simulink model "xeth"  (R2018a)
settings: Solver=VariableStepAuto  StartTime=0.0  StopTime=inf  RelTol=1e-3  EnableMultiTasking=on
undefined symbols (not defined in the file or in its folder): Part1, Part2, Part3, part4, RootGround, RootPart, taygap, xeth
libraries: mblibv1 x23, simulink x5
settings Model: Creator=phamn  LastModifiedBy=phamn
settings OptimizationCC: LifeSpan=inf
settings DebuggingCC: SFUnexpectedBacktrackingDiag=warning  SFNoUnconditionalDefaultTransitionDiag=warning  SFExecutionAtInitializationDiag=none
settings CodeAppCC: StateflowObjectComments=on
settings GRTTargetCC: TargetLangStandard=C89/C90 (ANSI)
settings ConfigComp: CovMetricSettings=dw  CovHtmlReporting=on  CovSaveCumulativeToWorkspaceVar=on  CovSaveSingleToWorkspaceVar=on  CovExternalEMLEnable=off
settings SimscapeCC: SimscapeNormalizeSystem=off
settings SimMechanicsCC: VisOnUpdateDiagram=on  VisDuringSimulation=on

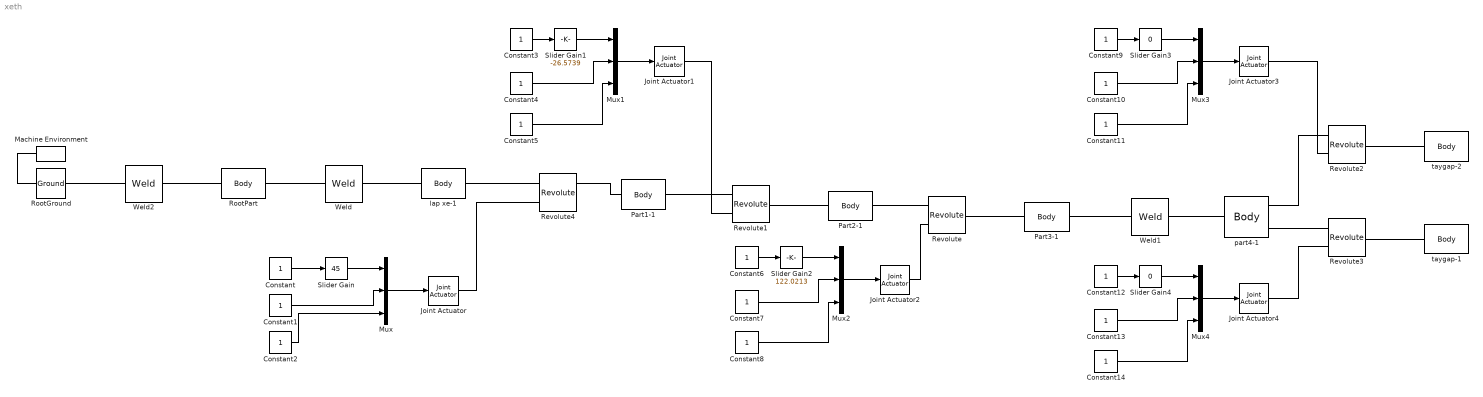
== system xeth ==
  Constant{,1..14} (15 alike) : Constant
  Joint Actuator{,1..4} (5 alike) : mblibv1/Sensors &  Actuators/Joint Actuator  UpdateFromCAD=off  PhysicalDomain=Mechanical  PortType=blob  ActuationStyle=Motion  AngleUnits=deg  ArcVelocityUnits=deg/s  ArcAccelerationUnits=deg/s^2  CoordPositionUnits=m  VelocityUnits=m/s  AccelerationUnits=m/s^2  ForceUnits=N  TorqueUnits=N*m  ActiveIO=on  Width=3  DialogClass=MechanicalActuatorBlock  Primitive=R1  ReferenceFrame=Absolute (World)
      settings: SourceProductName=Simscape  SourceProductBaseCode=SS
  Machine Environment : mblibv1/Bodies/Machine Environment  PortType=env  PhysicalDomain=Mechanical  DialogTemplateClass=MECH.MachineEnvironment  SyncWhenCopied=off  Gravity=[0 -9.81 0]  GravityUnits=m/s^2  GravityAsSignal=off  Dimensionality=Auto-detect  AnalysisType=Forward dynamics  LinearAssemblyTolerance=1e-3  LinearAssemblyToleranceUnits=m  AngularAssemblyTolerance=1e-3  AngularAssemblyToleranceUnits=rad  ConstraintSolverType=Stabilizing  ConstraintRelTolerance=1e-4  ConstraintAbsTolerance=1e-4  UseRobustSingularityHandling=off  RedundancyAnalysisToleranceType=Automatically select tolerance  RedundancyAnalysisTolerance=1e-14  StatePerturbationType=Fixed  PerturbationSize=1e-5  VisualizeMachine=on  BodyVisualizationType=Use model default body geometries  BodyColorSelMode=Use model default  DefaultBodyColor=[1 0 0]
      settings: SourceProductName=Simscape  SourceProductBaseCode=SS
  Mux{,1..4} (5 alike) : Mux  Inputs=3
  Part1-1 : mblibv1/Bodies/Body  LConnTagsString=CS3  RConnTagsString=CS2  UpdateFromCAD=on  PMImportedID=Part1-1  DialogClass=MechanicalBodyBlock  Mass=0.333703  MassUnits=kg  InertiaUnits=kg*m^2  Inertia=[0.00102628,0.000168229,6.01067e-10;0.000168229,0.000347488,-1.43807e-10;6.01067e-10,-1.43807e-10,0.000952025]  Shape=Cylinder  ShapeDims=[1 1]  ShapeUnits=m  ShapeUse=false  Density=1  DensityUnits=kg/m^3  DensityUse=false  GraphicsMode=GFXFILE  GraphicsFileName=xeth - Part1-1.STL  BodyColorSelMode=COLORPALETTE  BodyColor=[0.690196;0.658824;0.639216]  AttachedToCS=CS1  CG=Right$CG$[-0.0199579 0.0681608 0.0476382]$WORLD$WORLD$m$[-0.547791 0 0.836615;0 1 0;-0.836615 0 -0.547791]$3x3 Transform$rad$WORLD$false$Part1-1::CG(AUTOGEN)  WorkingFrames=Right$CS1$[-0.00787331 0.16628 0.0660944]$WORLD$WORLD$m$[-0.547791 0 0.836615;0 1 0;-0.836615 0 -0.547791]$3x3 Transform$rad$WORLD$false$Part1-1::CS1(AUTOGEN)#Right$CS2$[0.0109505 0.16628 0.0537691]$WORLD$WORLD$m$[1 0 0;0 1 0;0 0 1]$3x3 Transform$rad$WORLD$true$Part1-1:-:Part2-1::Part1-1(AUTOGEN)#Left$CS3$[-0.024307 0.02628 0.0409959]$WORLD$WORLD$m$[1 0 0;0 1 0;0 0 1]$3x3 Transform$rad$WORLD$true$Part1-1:-:lap xe-1::Part1-1(AUTOGEN)  CGPos=[-0.0199579 0.0681608 0.0476382]  CGRot=[-0.547791 0 0.836615;0 1 0;-0.836615 0 -0.547791]  CS0Pos=[]  CS0Rot=[]  CS1Pos=[-0.00787331 0.16628 0.0660944]  CS1Rot=[-0.547791 0 0.836615;0 1 0;-0.836615 0 -0.547791]  CS2Pos=[0.0109505 0.16628 0.0537691]  CS2Rot=[1 0 0;0 1 0;0 0 1]  CS3Pos=[-0.024307 0.02628 0.0409959]  CS3Rot=[1 0 0;0 1 0;0 0 1]  CS4Pos=[]  CS4Rot=[]  CS5Pos=[]  CS5Rot=[]  CS6Pos=[]  CS6Rot=[]  CS7Pos=[]  CS7Rot=[]  CS8Pos=[]  CS8Rot=[]  CS9Pos=[]  CS9Rot=[]  CS10Pos=[]  CS10Rot=[]  CS11Pos=[]  CS11Rot=[]  CS12Pos=[]  CS12Rot=[]  CS13Pos=[]  CS13Rot=[]  CS14Pos=[]  CS14Rot=[]  CS15Pos=[]  CS15Rot=[]  CS16Pos=[]  CS16Rot=[]  CS17Pos=[]  CS17Rot=[]  CS18Pos=[]  CS18Rot=[]  CS19Pos=[]  CS19Rot=[]  CS20Pos=[]  CS20Rot=[]
      settings: SourceProductName=Simscape  SourceProductBaseCode=SS
  Part2-1 : mblibv1/Bodies/Body  LConnTagsString=CS3  RConnTagsString=CS2  UpdateFromCAD=on  PMImportedID=Part2-1  DialogClass=MechanicalBodyBlock  Mass=0.215174  MassUnits=kg  InertiaUnits=kg*m^2  Inertia=[9.19526e-05,0,0;0,0.000457732,0;0,0,0.000463125]  Shape=Cylinder  ShapeDims=[1 1]  ShapeUnits=m  ShapeUse=false  Density=1  DensityUnits=kg/m^3  DensityUse=false  GraphicsMode=GFXFILE  GraphicsFileName=xeth - Part2-1.STL  BodyColorSelMode=COLORPALETTE  BodyColor=[0.690196;0.658824;0.639216]  AttachedToCS=CS1  CG=Right$CG$[0.0142867 0.159718 0.0999384]$WORLD$WORLD$m$[0.540722 0.836615 0.0877165;-0.160128 0 0.987096;0.82582 -0.547791 0.133965]$3x3 Transform$rad$WORLD$false$Part2-1::CG(AUTOGEN)  WorkingFrames=Right$CS1$[0.059717 0.146264 0.169322]$WORLD$WORLD$m$[0.540722 0.836615 0.0877165;-0.160128 0 0.987096;0.82582 -0.547791 0.133965]$3x3 Transform$rad$WORLD$false$Part2-1::CS1(AUTOGEN)#Right$CS2$[0.0722662 0.146264 0.161105]$WORLD$WORLD$m$[1 0 0;0 1 0;0 0 1]$3x3 Transform$rad$WORLD$true$Part2-1:-:Part3-1::Part2-1(AUTOGEN)#Left$CS3$[0.0109505 0.16628 0.0537691]$WORLD$WORLD$m$[1 0 0;0 1 0;0 0 1]$3x3 Transform$rad$WORLD$true$Part1-1:-:Part2-1::Part2-1(AUTOGEN)  CGPos=[0.0142867 0.159718 0.0999384]  CGRot=[0.540722 0.836615 0.0877165;-0.160128 0 0.987096;0.82582 -0.547791 0.133965]  CS0Pos=[]  CS0Rot=[]  CS1Pos=[0.059717 0.146264 0.169322]  CS1Rot=[0.540722 0.836615 0.0877165;-0.160128 0 0.987096;0.82582 -0.547791 0.133965]  CS2Pos=[0.0722662 0.146264 0.161105]  CS2Rot=[1 0 0;0 1 0;0 0 1]  CS3Pos=[0.0109505 0.16628 0.0537691]  CS3Rot=[1 0 0;0 1 0;0 0 1]  CS4Pos=[]  CS4Rot=[]  CS5Pos=[]  CS5Rot=[]  CS6Pos=[]  CS6Rot=[]  CS7Pos=[]  CS7Rot=[]  CS8Pos=[]  CS8Rot=[]  CS9Pos=[]  CS9Rot=[]  CS10Pos=[]  CS10Rot=[]  CS11Pos=[]  CS11Rot=[]  CS12Pos=[]  CS12Rot=[]  CS13Pos=[]  CS13Rot=[]  CS14Pos=[]  CS14Rot=[]  CS15Pos=[]  CS15Rot=[]  CS16Pos=[]  CS16Rot=[]  CS17Pos=[]  CS17Rot=[]  CS18Pos=[]  CS18Rot=[]  CS19Pos=[]  CS19Rot=[]  CS20Pos=[]  CS20Rot=[]
      settings: SourceProductName=Simscape  SourceProductBaseCode=SS
  Part3-1 : mblibv1/Bodies/Body  LConnTagsString=CS2  RConnTagsString=CS3  UpdateFromCAD=on  PMImportedID=Part3-1  DialogClass=MechanicalBodyBlock  Mass=0.0734899  MassUnits=kg  InertiaUnits=kg*m^2  Inertia=[1.76028e-05,0,0;0,6.41753e-05,1.2079e-11;0,1.2079e-11,5.96726e-05]  Shape=Cylinder  ShapeDims=[1 1]  ShapeUnits=m  ShapeUse=false  Density=1  DensityUnits=kg/m^3  DensityUse=false  GraphicsMode=GFXFILE  GraphicsFileName=xeth - Part3-1.STL  BodyColorSelMode=COLORPALETTE  BodyColor=[0.690196;0.658824;0.639216]  AttachedToCS=CS1  CG=Right$CG$[0.0671334 0.141842 0.180649]$WORLD$WORLD$m$[0.520722 0.836615 0.17007;-0.310465 0 0.950585;0.795274 -0.547791 0.25974]$3x3 Transform$rad$WORLD$false$Part3-1::CG(AUTOGEN)  WorkingFrames=Right$CS1$[0.0987711 0.122979 0.228967]$WORLD$WORLD$m$[0.520722 0.836615 0.17007;-0.310465 0 0.950585;0.795274 -0.547791 0.25974]$3x3 Transform$rad$WORLD$false$Part3-1::CS1(AUTOGEN)#Left$CS2$[0.0722662 0.146264 0.161105]$WORLD$WORLD$m$[1 0 0;0 1 0;0 0 1]$3x3 Transform$rad$WORLD$true$Part2-1:-:Part3-1::Part3-1(AUTOGEN)#Right$CS3$[0.0816912 0.138694 0.221137]$WORLD$WORLD$m$[1 0 0;0 1 0;0 0 1]$3x3 Transform$rad$WORLD$true$Part3-1:-:part4-1::Part3-1(AUTOGEN)  CGPos=[0.0671334 0.141842 0.180649]  CGRot=[0.520722 0.836615 0.17007;-0.310465 0 0.950585;0.795274 -0.547791 0.25974]  CS0Pos=[]  CS0Rot=[]  CS1Pos=[0.0987711 0.122979 0.228967]  CS1Rot=[0.520722 0.836615 0.17007;-0.310465 0 0.950585;0.795274 -0.547791 0.25974]  CS2Pos=[0.0722662 0.146264 0.161105]  CS2Rot=[1 0 0;0 1 0;0 0 1]  CS3Pos=[0.0816912 0.138694 0.221137]  CS3Rot=[1 0 0;0 1 0;0 0 1]  CS4Pos=[]  CS4Rot=[]  CS5Pos=[]  CS5Rot=[]  CS6Pos=[]  CS6Rot=[]  CS7Pos=[]  CS7Rot=[]  CS8Pos=[]  CS8Rot=[]  CS9Pos=[]  CS9Rot=[]  CS10Pos=[]  CS10Rot=[]  CS11Pos=[]  CS11Rot=[]  CS12Pos=[]  CS12Rot=[]  CS13Pos=[]  CS13Rot=[]  CS14Pos=[]  CS14Rot=[]  CS15Pos=[]  CS15Rot=[]  CS16Pos=[]  CS16Rot=[]  CS17Pos=[]  CS17Rot=[]  CS18Pos=[]  CS18Rot=[]  CS19Pos=[]  CS19Rot=[]  CS20Pos=[]  CS20Rot=[]
      settings: SourceProductName=Simscape  SourceProductBaseCode=SS
  Revolute : mblibv1/Joints/Revolute  LConnTagsString=__newl0|SA1  RConnTagsString=__newr0  UpdateFromCAD=on  PMImportedID=Part2-1:-:Part3-1  NumSAPorts=1  CutJoint=off  MarkAsCut=off  Primitives=prismatic  PrimitiveProps=R1$World$[0.836615,0,-0.547791]$revolute  DialogClass=JointBlock  R1Axis=[0.836615,0,-0.547791]
      settings: SourceProductName=Simscape  SourceProductBaseCode=SS
  Revolute1 : mblibv1/Joints/Revolute  LConnTagsString=__newl0|SA1  RConnTagsString=__newr0  UpdateFromCAD=on  PMImportedID=Part1-1:-:Part2-1  NumSAPorts=1  CutJoint=off  MarkAsCut=off  Primitives=prismatic  PrimitiveProps=R1$World$[0.836615,0,-0.547791]$revolute  DialogClass=JointBlock  R1Axis=[0.836615,0,-0.547791]
      settings: SourceProductName=Simscape  SourceProductBaseCode=SS
  Revolute2 : mblibv1/Joints/Revolute  LConnTagsString=__newl0|SA1  RConnTagsString=__newr0  UpdateFromCAD=on  PMImportedID=part4-1:-:taygap-2  NumSAPorts=1  CutJoint=off  MarkAsCut=off  Primitives=prismatic  PrimitiveProps=R1$World$[0.17007,0.950585,0.25974]$revolute  DialogClass=JointBlock  R1Axis=[0.17007,0.950585,0.25974]
      settings: SourceProductName=Simscape  SourceProductBaseCode=SS
  Revolute3 : mblibv1/Joints/Revolute  LConnTagsString=__newl0|SA1  RConnTagsString=__newr0  UpdateFromCAD=on  PMImportedID=part4-1:-:taygap-1  NumSAPorts=1  CutJoint=off  MarkAsCut=off  Primitives=prismatic  PrimitiveProps=R1$World$[0.17007,0.950585,0.25974]$revolute  DialogClass=JointBlock  R1Axis=[0.17007,0.950585,0.25974]
      settings: SourceProductName=Simscape  SourceProductBaseCode=SS
  Revolute4 : mblibv1/Joints/Revolute  LConnTagsString=__newl0|SA1  RConnTagsString=__newr0|SA1  UpdateFromCAD=on  PMImportedID=Part1-1:-:lap xe-1  NumSAPorts=2  CutJoint=off  MarkAsCut=off  Primitives=prismatic  PrimitiveProps=R1$World$[0,1,0]$revolute  DialogClass=JointBlock  R1Axis=[0,1,0]
      settings: SourceProductName=Simscape  SourceProductBaseCode=SS
  RootGround : mblibv1/Bodies/Ground  UpdateFromCAD=on  PMImportedID=RootGround  LeftPortType=env  RightPortType=workingframe  PhysicalDomain=Mechanical  DialogClass=GroundBlock  CoordPosition=[-0.0268327,0.0402031,0.0611544]  CoordPositionUnits=m  StateVectorMgrId=0  MachineId=[1 0]  ShowEnvPort=on  ParameterChecksum=[4032550197, 4140926949, 1037704833, 3004748647]  TopologyChecksum=[501219954, 3028778896, 2402402702, 776814038]
      settings: SourceProductName=Simscape  SourceProductBaseCode=SS
  RootPart : mblibv1/Bodies/Body  LConnTagsString=CS3  RConnTagsString=CS2  UpdateFromCAD=on  PMImportedID=xeth/RootPart  DialogClass=MechanicalBodyBlock  Mass=0  MassUnits=kg  InertiaUnits=kg*m^2  Inertia=[0,0,0;0,0,0;0,0,0]  Shape=Cylinder  ShapeDims=[1 1]  ShapeUnits=m  ShapeUse=false  Density=1  DensityUnits=kg/m^3  DensityUse=false  GraphicsMode=MACHINE_DEFAULT  BodyColorSelMode=MACHINE_DEFAULT  BodyColor=[1;0;0]  AttachedToCS=CS1  CG=Right$CG$[-0.0268327 0.0402031 0.0611544]$WORLD$WORLD$m$[1 0 0;0 1 0;0 0 1]$3x3 Transform$rad$WORLD$false$xeth/RootPart::CG(AUTOGEN)  WorkingFrames=Right$CS1$[0 0 0]$WORLD$WORLD$m$[1 0 0;0 1 0;0 0 1]$3x3 Transform$rad$WORLD$false$xeth/RootPart::CS1(AUTOGEN)#Right$CS2$[-0.0530982 -0.0169014 0.0409959]$WORLD$WORLD$m$[1 0 0;0 1 0;0 0 1]$3x3 Transform$rad$WORLD$true$lap xe-1:-:xeth/RootPart::xeth/RootPart(AUTOGEN)#Left$CS3$[-0.0268327 0.0402031 0.0611544]$WORLD$WORLD$m$[1 0 0;0 1 0;0 0 1]$3x3 Transform$rad$WORLD$true$RootGround:-:xeth/RootPart::xeth/RootPart(AUTOGEN)  CGPos=[-0.0268327 0.0402031 0.0611544]  CGRot=[1 0 0;0 1 0;0 0 1]  CS0Pos=[]  CS0Rot=[]  CS1Pos=[0 0 0]  CS1Rot=[1 0 0;0 1 0;0 0 1]  CS2Pos=[-0.0530982 -0.0169014 0.0409959]  CS2Rot=[1 0 0;0 1 0;0 0 1]  CS3Pos=[-0.0268327 0.0402031 0.0611544]  CS3Rot=[1 0 0;0 1 0;0 0 1]  CS4Pos=[]  CS4Rot=[]  CS5Pos=[]  CS5Rot=[]  CS6Pos=[]  CS6Rot=[]  CS7Pos=[]  CS7Rot=[]  CS8Pos=[]  CS8Rot=[]  CS9Pos=[]  CS9Rot=[]  CS10Pos=[]  CS10Rot=[]  CS11Pos=[]  CS11Rot=[]  CS12Pos=[]  CS12Rot=[]  CS13Pos=[]  CS13Rot=[]  CS14Pos=[]  CS14Rot=[]  CS15Pos=[]  CS15Rot=[]  CS16Pos=[]  CS16Rot=[]  CS17Pos=[]  CS17Rot=[]  CS18Pos=[]  CS18Rot=[]  CS19Pos=[]  CS19Rot=[]  CS20Pos=[]  CS20Rot=[]
      settings: SourceProductName=Simscape  SourceProductBaseCode=SS
  Slider Gain : simulink/Math Operations/Slider Gain  gain=45  low=-180  high=240
  Slider Gain1 : simulink/Math Operations/Slider Gain  gain=-26.5739  low=-150  high=150
  Slider Gain2 : simulink/Math Operations/Slider Gain  gain=122.0213  low=-150  high=150
  Slider Gain3 : simulink/Math Operations/Slider Gain  gain=0  low=0  high=90
  Slider Gain4 : simulink/Math Operations/Slider Gain  gain=0  low=-90  high=0
  Weld : mblibv1/Joints/Weld  LConnTagsString=__newl0  RConnTagsString=__newr0  UpdateFromCAD=on  PMImportedID=lap xe-1:-:xeth/RootPart  NumSAPorts=0  CutJoint=off  MarkAsCut=off  Primitives=weld  PrimitiveProps=W$WORLD$[0.57735,0.57735,0.57735]$weld  DialogClass=JointBlock  WAxis=[0.57735,0.57735,0.57735]
      settings: SourceProductName=Simscape  SourceProductBaseCode=SS
  Weld1 : mblibv1/Joints/Weld  LConnTagsString=__newl0  RConnTagsString=__newr0  UpdateFromCAD=on  PMImportedID=Part3-1:-:part4-1  NumSAPorts=0  CutJoint=off  MarkAsCut=off  Primitives=weld  PrimitiveProps=W$WORLD$[0.57735,0.57735,0.57735]$weld  DialogClass=JointBlock  WAxis=[0.57735,0.57735,0.57735]
      settings: SourceProductName=Simscape  SourceProductBaseCode=SS
  Weld2 : mblibv1/Joints/Weld  LConnTagsString=__newl0  RConnTagsString=__newr0  UpdateFromCAD=on  PMImportedID=RootGround:-:xeth/RootPart  NumSAPorts=0  CutJoint=off  MarkAsCut=off  Primitives=weld  PrimitiveProps=W$WORLD$[0.57735,0.57735,0.57735]$weld  DialogClass=JointBlock  WAxis=[0.57735,0.57735,0.57735]
      settings: SourceProductName=Simscape  SourceProductBaseCode=SS
  lap xe-1 : mblibv1/Bodies/Body  LConnTagsString=CS2  RConnTagsString=CS3  UpdateFromCAD=on  PMImportedID=lap xe-1  DialogClass=MechanicalBodyBlock  Mass=0.767257  MassUnits=kg  InertiaUnits=kg*m^2  Inertia=[0.00251277,4.31285e-05,0;4.31285e-05,0.00516616,0;0,0,0.00330555]  Shape=Cylinder  ShapeDims=[1 1]  ShapeUnits=m  ShapeUse=false  Density=1  DensityUnits=kg/m^3  DensityUse=false  GraphicsMode=GFXFILE  GraphicsFileName=xeth - lap xe-1.STL  BodyColorSelMode=COLORPALETTE  BodyColor=[0.752941;0.752941;0.752941]  AttachedToCS=CS1  CG=Right$CG$[-0.0530982 -0.0169014 0.0409959]$WORLD$WORLD$m$[1 0 0;0 1 0;0 0 1]$3x3 Transform$rad$WORLD$false$lap xe-1::CG(AUTOGEN)  WorkingFrames=Right$CS1$[-0.0981233 -0.101598 -0.114716]$WORLD$WORLD$m$[1 0 0;0 1 0;0 0 1]$3x3 Transform$rad$WORLD$false$lap xe-1::CS1(AUTOGEN)#Left$CS2$[-0.0530982 -0.0169014 0.0409959]$WORLD$WORLD$m$[1 0 0;0 1 0;0 0 1]$3x3 Transform$rad$WORLD$true$lap xe-1:-:xeth/RootPart::lap xe-1(AUTOGEN)#Right$CS3$[-0.024307 0.02628 0.0409959]$WORLD$WORLD$m$[1 0 0;0 1 0;0 0 1]$3x3 Transform$rad$WORLD$true$Part1-1:-:lap xe-1::lap xe-1(AUTOGEN)  CGPos=[-0.0530982 -0.0169014 0.0409959]  CGRot=[1 0 0;0 1 0;0 0 1]  CS0Pos=[]  CS0Rot=[]  CS1Pos=[-0.0981233 -0.101598 -0.114716]  CS1Rot=[1 0 0;0 1 0;0 0 1]  CS2Pos=[-0.0530982 -0.0169014 0.0409959]  CS2Rot=[1 0 0;0 1 0;0 0 1]  CS3Pos=[-0.024307 0.02628 0.0409959]  CS3Rot=[1 0 0;0 1 0;0 0 1]  CS4Pos=[]  CS4Rot=[]  CS5Pos=[]  CS5Rot=[]  CS6Pos=[]  CS6Rot=[]  CS7Pos=[]  CS7Rot=[]  CS8Pos=[]  CS8Rot=[]  CS9Pos=[]  CS9Rot=[]  CS10Pos=[]  CS10Rot=[]  CS11Pos=[]  CS11Rot=[]  CS12Pos=[]  CS12Rot=[]  CS13Pos=[]  CS13Rot=[]  CS14Pos=[]  CS14Rot=[]  CS15Pos=[]  CS15Rot=[]  CS16Pos=[]  CS16Rot=[]  CS17Pos=[]  CS17Rot=[]  CS18Pos=[]  CS18Rot=[]  CS19Pos=[]  CS19Rot=[]  CS20Pos=[]  CS20Rot=[]
      settings: SourceProductName=Simscape  SourceProductBaseCode=SS
  part4-1 : mblibv1/Bodies/Body  LConnTagsString=CS4  RConnTagsString=CS2|CS3  UpdateFromCAD=on  PMImportedID=part4-1  DialogClass=MechanicalBodyBlock  Mass=0.0116579  MassUnits=kg  InertiaUnits=kg*m^2  Inertia=[8.25813e-07,0,0;0,3.44208e-06,0;0,0,3.16008e-06]  Shape=Cylinder  ShapeDims=[1 1]  ShapeUnits=m  ShapeUse=false  Density=1  DensityUnits=kg/m^3  DensityUse=false  GraphicsMode=GFXFILE  GraphicsFileName=xeth - part4-1.STL  BodyColorSelMode=COLORPALETTE  BodyColor=[0.792157;0.819608;0.933333]  AttachedToCS=CS1  CG=Right$CG$[0.0985401 0.123117 0.228615]$WORLD$WORLD$m$[0.520722 0.17007 -0.836615;-0.310465 0.950585 0;0.795274 0.25974 0.547791]$3x3 Transform$rad$WORLD$false$part4-1::CG(AUTOGEN)  WorkingFrames=Right$CS1$[0.108325 0.115179 0.243558]$WORLD$WORLD$m$[0.520722 0.17007 -0.836615;-0.310465 0.950585 0;0.795274 0.25974 0.547791]$3x3 Transform$rad$WORLD$false$part4-1::CS1(AUTOGEN)#Right$CS2$[0.117371 0.118981 0.239119]$WORLD$WORLD$m$[1 0 0;0 1 0;0 0 1]$3x3 Transform$rad$WORLD$true$part4-1:-:taygap-2::part4-1(AUTOGEN)#Right$CS3$[0.100639 0.118981 0.250075]$WORLD$WORLD$m$[1 0 0;0 1 0;0 0 1]$3x3 Transform$rad$WORLD$true$part4-1:-:taygap-1::part4-1(AUTOGEN)#Left$CS4$[0.0816912 0.138694 0.221137]$WORLD$WORLD$m$[1 0 0;0 1 0;0 0 1]$3x3 Transform$rad$WORLD$true$Part3-1:-:part4-1::part4-1(AUTOGEN)  CGPos=[0.0985401 0.123117 0.228615]  CGRot=[0.520722 0.17007 -0.836615;-0.310465 0.950585 0;0.795274 0.25974 0.547791]  CS0Pos=[]  CS0Rot=[]  CS1Pos=[0.108325 0.115179 0.243558]  CS1Rot=[0.520722 0.17007 -0.836615;-0.310465 0.950585 0;0.795274 0.25974 0.547791]  CS2Pos=[0.117371 0.118981 0.239119]  CS2Rot=[1 0 0;0 1 0;0 0 1]  CS3Pos=[0.100639 0.118981 0.250075]  CS3Rot=[1 0 0;0 1 0;0 0 1]  CS4Pos=[0.0816912 0.138694 0.221137]  CS4Rot=[1 0 0;0 1 0;0 0 1]  CS5Pos=[]  CS5Rot=[]  CS6Pos=[]  CS6Rot=[]  CS7Pos=[]  CS7Rot=[]  CS8Pos=[]  CS8Rot=[]  CS9Pos=[]  CS9Rot=[]  CS10Pos=[]  CS10Rot=[]  CS11Pos=[]  CS11Rot=[]  CS12Pos=[]  CS12Rot=[]  CS13Pos=[]  CS13Rot=[]  CS14Pos=[]  CS14Rot=[]  CS15Pos=[]  CS15Rot=[]  CS16Pos=[]  CS16Rot=[]  CS17Pos=[]  CS17Rot=[]  CS18Pos=[]  CS18Rot=[]  CS19Pos=[]  CS19Rot=[]  CS20Pos=[]  CS20Rot=[]
      settings: SourceProductName=Simscape  SourceProductBaseCode=SS
  taygap-1 : mblibv1/Bodies/Body  LConnTagsString=CS2  UpdateFromCAD=on  PMImportedID=taygap-1  DialogClass=MechanicalBodyBlock  Mass=0.00223614  MassUnits=kg  InertiaUnits=kg*m^2  Inertia=[7.89446e-08,0,6.55068e-08;0,8.91507e-07,0;6.55068e-08,0,8.16331e-07]  Shape=Cylinder  ShapeDims=[1 1]  ShapeUnits=m  ShapeUse=false  Density=1  DensityUnits=kg/m^3  DensityUse=false  GraphicsMode=GFXFILE  GraphicsFileName=xeth - taygap-1.STL  BodyColorSelMode=COLORPALETTE  BodyColor=[0.792157;0.819608;0.933333]  AttachedToCS=CS1  CG=Right$CG$[0.106946 0.114475 0.268213]$WORLD$WORLD$m$[0.428244 -0.17007 0.887515;-0.308684 -0.950585 -0.0332095;0.849306 -0.25974 -0.45958]$3x3 Transform$rad$WORLD$false$taygap-1::CG(AUTOGEN)  WorkingFrames=Right$CS1$[0.126799 0.104219 0.292747]$WORLD$WORLD$m$[0.428244 -0.17007 0.887515;-0.308684 -0.950585 -0.0332095;0.849306 -0.25974 -0.45958]$3x3 Transform$rad$WORLD$false$taygap-1::CS1(AUTOGEN)#Left$CS2$[0.100639 0.118981 0.250075]$WORLD$WORLD$m$[1 0 0;0 1 0;0 0 1]$3x3 Transform$rad$WORLD$true$part4-1:-:taygap-1::taygap-1(AUTOGEN)  CGPos=[0.106946 0.114475 0.268213]  CGRot=[0.428244 -0.17007 0.887515;-0.308684 -0.950585 -0.0332095;0.849306 -0.25974 -0.45958]  CS0Pos=[]  CS0Rot=[]  CS1Pos=[0.126799 0.104219 0.292747]  CS1Rot=[0.428244 -0.17007 0.887515;-0.308684 -0.950585 -0.0332095;0.849306 -0.25974 -0.45958]  CS2Pos=[0.100639 0.118981 0.250075]  CS2Rot=[1 0 0;0 1 0;0 0 1]  CS3Pos=[]  CS3Rot=[]  CS4Pos=[]  CS4Rot=[]  CS5Pos=[]  CS5Rot=[]  CS6Pos=[]  CS6Rot=[]  CS7Pos=[]  CS7Rot=[]  CS8Pos=[]  CS8Rot=[]  CS9Pos=[]  CS9Rot=[]  CS10Pos=[]  CS10Rot=[]  CS11Pos=[]  CS11Rot=[]  CS12Pos=[]  CS12Rot=[]  CS13Pos=[]  CS13Rot=[]  CS14Pos=[]  CS14Rot=[]  CS15Pos=[]  CS15Rot=[]  CS16Pos=[]  CS16Rot=[]  CS17Pos=[]  CS17Rot=[]  CS18Pos=[]  CS18Rot=[]  CS19Pos=[]  CS19Rot=[]  CS20Pos=[]  CS20Rot=[]
      settings: SourceProductName=Simscape  SourceProductBaseCode=SS
  taygap-2 : mblibv1/Bodies/Body  LConnTagsString=CS2  UpdateFromCAD=on  PMImportedID=taygap-2  DialogClass=MechanicalBodyBlock  Mass=0.00223614  MassUnits=kg  InertiaUnits=kg*m^2  Inertia=[7.89446e-08,0,6.55068e-08;0,8.91507e-07,0;6.55068e-08,0,8.16331e-07]  Shape=Cylinder  ShapeDims=[1 1]  ShapeUnits=m  ShapeUse=false  Density=1  DensityUnits=kg/m^3  DensityUse=false  GraphicsMode=GFXFILE  GraphicsFileName=xeth - taygap-2.STL  BodyColorSelMode=COLORPALETTE  BodyColor=[0.792157;0.819608;0.933333]  AttachedToCS=CS1  CG=Right$CG$[0.127065 0.114308 0.25565]$WORLD$WORLD$m$[0.362451 0.17007 -0.916354;-0.305444 0.950585 0.0556086;0.88053 0.25974 0.396488]$3x3 Transform$rad$WORLD$false$taygap-2::CG(AUTOGEN)  WorkingFrames=Right$CS1$[0.13272 0.104752 0.286921]$WORLD$WORLD$m$[0.362451 0.17007 -0.916354;-0.305444 0.950585 0.0556086;0.88053 0.25974 0.396488]$3x3 Transform$rad$WORLD$false$taygap-2::CS1(AUTOGEN)#Left$CS2$[0.117371 0.118981 0.239119]$WORLD$WORLD$m$[1 0 0;0 1 0;0 0 1]$3x3 Transform$rad$WORLD$true$part4-1:-:taygap-2::taygap-2(AUTOGEN)  CGPos=[0.127065 0.114308 0.25565]  CGRot=[0.362451 0.17007 -0.916354;-0.305444 0.950585 0.0556086;0.88053 0.25974 0.396488]  CS0Pos=[]  CS0Rot=[]  CS1Pos=[0.13272 0.104752 0.286921]  CS1Rot=[0.362451 0.17007 -0.916354;-0.305444 0.950585 0.0556086;0.88053 0.25974 0.396488]  CS2Pos=[0.117371 0.118981 0.239119]  CS2Rot=[1 0 0;0 1 0;0 0 1]  CS3Pos=[]  CS3Rot=[]  CS4Pos=[]  CS4Rot=[]  CS5Pos=[]  CS5Rot=[]  CS6Pos=[]  CS6Rot=[]  CS7Pos=[]  CS7Rot=[]  CS8Pos=[]  CS8Rot=[]  CS9Pos=[]  CS9Rot=[]  CS10Pos=[]  CS10Rot=[]  CS11Pos=[]  CS11Rot=[]  CS12Pos=[]  CS12Rot=[]  CS13Pos=[]  CS13Rot=[]  CS14Pos=[]  CS14Rot=[]  CS15Pos=[]  CS15Rot=[]  CS16Pos=[]  CS16Rot=[]  CS17Pos=[]  CS17Rot=[]  CS18Pos=[]  CS18Rot=[]  CS19Pos=[]  CS19Rot=[]  CS20Pos=[]  CS20Rot=[]
      settings: SourceProductName=Simscape  SourceProductBaseCode=SS
  wires:
  Constant/1 -> Slider Gain/1
  Constant1/1 -> Mux/2
  Constant2/1 -> Mux/3
  Constant3/1 -> Slider Gain1/1
  Slider Gain1/1 -> Mux1/1
  Constant4/1 -> Mux1/2
  Constant5/1 -> Mux1/3
  Mux1/1 -> Joint Actuator1/1
  Constant6/1 -> Slider Gain2/1
  Slider Gain2/1 -> Mux2/1
  Constant7/1 -> Mux2/2
  Constant8/1 -> Mux2/3
  Mux2/1 -> Joint Actuator2/1
  Constant9/1 -> Slider Gain3/1
  Slider Gain3/1 -> Mux3/1
  Constant10/1 -> Mux3/2
  Constant11/1 -> Mux3/3
  Mux3/1 -> Joint Actuator3/1
  Constant12/1 -> Slider Gain4/1
  Slider Gain4/1 -> Mux4/1
  Constant13/1 -> Mux4/2
  Constant14/1 -> Mux4/3
  Mux4/1 -> Joint Actuator4/1
  Mux/1 -> Joint Actuator/1
  Slider Gain/1 -> Mux/1
  connections:
  RootPart/RConn1 -- Weld/LConn1
  Weld/RConn1 -- lap xe-1/LConn1
  Part2-1/RConn1 -- Revolute/LConn1
  Revolute/RConn1 -- Part3-1/LConn1
  Part1-1/RConn1 -- Revolute1/LConn1
  Revolute1/RConn1 -- Part2-1/LConn1
  part4-1/RConn1 -- Revolute2/LConn1
  Revolute2/RConn1 -- taygap-2/LConn1
  part4-1/RConn2 -- Revolute3/LConn1
  Revolute3/RConn1 -- taygap-1/LConn1
  Part3-1/RConn1 -- Weld1/LConn1
  Weld1/RConn1 -- part4-1/LConn1
  lap xe-1/RConn1 -- Revolute4/LConn1
  RootGround/RConn1 -- Weld2/LConn1
  Weld2/RConn1 -- RootPart/LConn1
  RootGround/LConn1 -- Machine Environment/RConn1
  Joint Actuator1/RConn1 -- Revolute1/LConn2
  Joint Actuator2/RConn1 -- Revolute/LConn2
  Joint Actuator3/RConn1 -- Revolute2/LConn2
  Joint Actuator4/RConn1 -- Revolute3/LConn2
  Joint Actuator/RConn1 -- Revolute4/LConn2
  Revolute4/RConn1 -- Part1-1/LConn1
